simulink model "qMultiply"  (R2018a)
settings: Solver=VariableStepAuto  StartTime=0.0  StopTime=10.0  RelTol=1e-3
libraries: vrlib x1
settings Model: Creator=henry  LastModifiedBy=henry

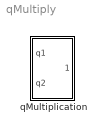
== system qMultiply ==
  qMultiplication : Subsystem  mask(Quaternion Multiplication){}
      mask help: This block performs the quaternion multiplication given two input quaternions.

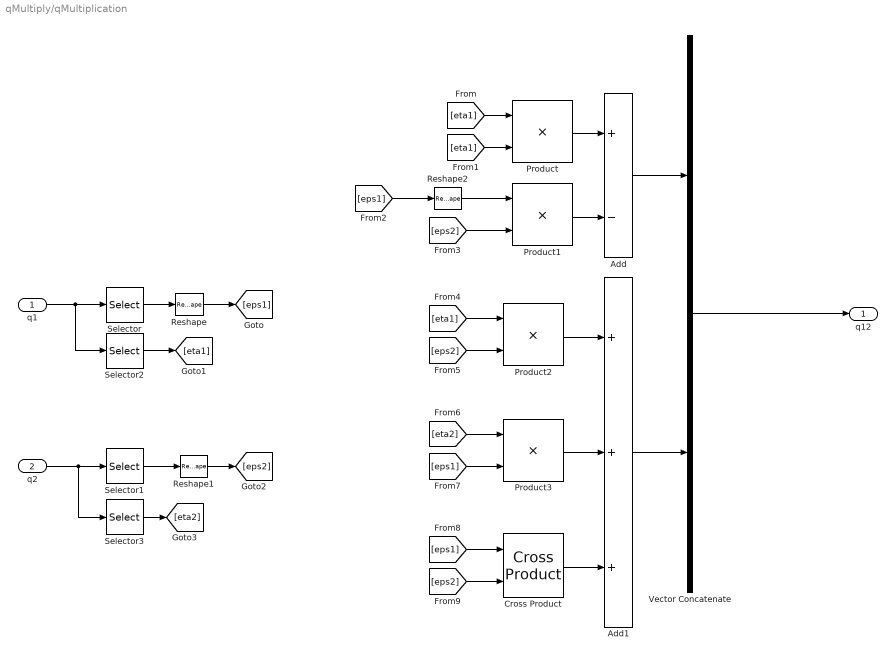
== system qMultiply/qMultiplication ==
  q1 : Inport
  q2 : Inport  Port=2
  Add : Sum  Inputs=+-
  Add1 : Sum  Inputs=+++
  Cross Product : vrlib/Utilities/Cross Product
      settings: SourceProductBaseCode=VR
  Product{,1..3} (4 alike) : Product
  Reshape : Reshape
  Reshape1 : Reshape
  Reshape2 : Reshape
  Selector : Selector  InputPortWidth=4  IndexOptions=Index vector (dialog)  Indices=[1:3]  OutputSizes=1
  Selector1 : Selector  InputPortWidth=4  IndexOptions=Index vector (dialog)  Indices=[1:3]  OutputSizes=1
  Selector2 : Selector  InputPortWidth=4  IndexOptions=Index vector (dialog)  Indices=4  OutputSizes=1
  Selector3 : Selector  InputPortWidth=4  IndexOptions=Index vector (dialog)  Indices=4  OutputSizes=1
  Vector Concatenate : Concatenate
  q12 : Outport
  wires:
  Selector3/1 -> [eta2]
  Product2/1 -> Add1/1
  Product/1 -> Add/1
  [eta1] -> Product2/1
  [eta1] -> Product/2
  Selector1/1 -> Reshape1/1
  Product3/1 -> Add1/2
  q1/1 -> Selector2/1, Selector/1
  Reshape2/1 -> Product1/1
  Selector2/1 -> [eta1]
  Reshape1/1 -> [eps2]
  Add/1 -> Vector Concatenate/1
  Cross Product/1 -> Add1/3
  [eps1] -> Reshape2/1
  q2/1 -> Selector3/1, Selector1/1
  [eta2] -> Product3/1
  [eta1] -> Product/1
  Vector Concatenate/1 -> q12/1
  Add1/1 -> Vector Concatenate/2
  Selector/1 -> Reshape/1
  [eps2] -> Product2/2
  [eps1] -> Product3/2
  Reshape/1 -> [eps1]
  [eps2] -> Cross Product/2
  Product1/1 -> Add/2
  [eps1] -> Cross Product/1
  [eps2] -> Product1/2
